simulink model "identificacion_auxV2018"  (R2018a)
settings: Solver=VariableStepAuto  StartTime=0.0  StopTime=100  RelTol=1e-3
libraries: simulink x1
settings Model: Creator=gamam  LastModifiedBy=chech
settings SolverCC: AlgebraicLoopSolver=LineSearch
settings DebuggingCC: AlgebraicLoopMsg=none

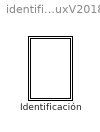
== system identificacion_auxV2018 ==
  Identificación : Subsystem

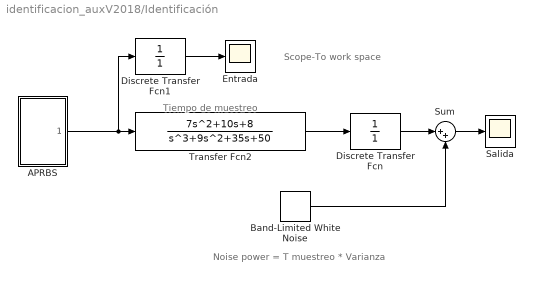
== system identificacion_auxV2018/Identificación ==
  note: Tiempo de muestreo
  note: Scope-To work space
  note: Noise power = T muestreo * Varianza
  APRBS : Subsystem
  Band-Limited White Noise : simulink/Sources/Band-Limited White Noise  Cov=[0.0001]  Ts=0.1  seed=[0]
  Discrete Transfer Fcn : DiscreteTransferFcn  Denominator=[1]  SampleTime=0.1
  Discrete Transfer Fcn1 : DiscreteTransferFcn  Denominator=[1]  SampleTime=0.1
  Entrada : Scope
  Salida : Scope
  Sum : Sum  Inputs=|++
  Transfer Fcn2 : TransferFcn  Numerator=[7 10 8]  Denominator=[1 9 35 50]
  wires:
  APRBS/1(u_ident) -> Transfer Fcn2/1, Discrete Transfer Fcn1/1
  Band-Limited White Noise/1 -> Sum/2
  Sum/1 -> Salida/1
  Transfer Fcn2/1 -> Discrete Transfer Fcn/1
  Discrete Transfer Fcn1/1 -> Entrada/1
  Discrete Transfer Fcn/1 -> Sum/1

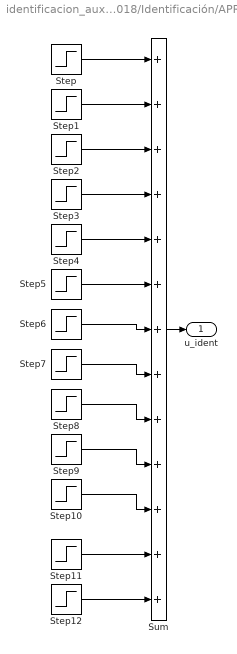
== system identificacion_auxV2018/Identificación/APRBS ==
  Step : Step  SampleTime=0
  Step1 : Step  Time=12  After=2  SampleTime=0
  Step10 : Step  Time=92  After=-3.5  SampleTime=0
  Step11 : Step  Time=95  After=1.8  SampleTime=0
  Step12 : Step  Time=98  SampleTime=0
  Step2 : Step  Time=21  After=2  SampleTime=0
  Step3 : Step  Time=29  After=-4  SampleTime=0
  Step4 : Step  Time=38  After=1+2.5  SampleTime=0
  Step5 : Step  Time=45  After=2.5  SampleTime=0
  Step6 : Step  Time=58  After=-3  SampleTime=0
  Step7 : Step  Time=68  After=0.5  SampleTime=0
  Step8 : Step  Time=72  After=-1.5  SampleTime=0
  Step9 : Step  Time=88  After=3  SampleTime=0
  Sum : Sum  Inputs=+++++++++++++
  u_ident : Outport  VectorParamsAs1DForOutWhenUnconnected=off
  wires:
  Sum/1 -> u_ident/1
  Step9/1 -> Sum/10
  Step6/1 -> Sum/7
  Step11/1 -> Sum/12
  Step4/1 -> Sum/5
  Step2/1 -> Sum/3
  Step/1 -> Sum/1
  Step5/1 -> Sum/6
  Step12/1 -> Sum/13
  Step3/1 -> Sum/4
  Step7/1 -> Sum/8
  Step1/1 -> Sum/2
  Step10/1 -> Sum/11
  Step8/1 -> Sum/9
